simulink model "chap2_2"  (Simulink 3.00)
settings: Solver=ode45  StartTime=0.0  StopTime=10.0  RelTol=1e-3
libraries: simulink3 x1, simulink_extras x1

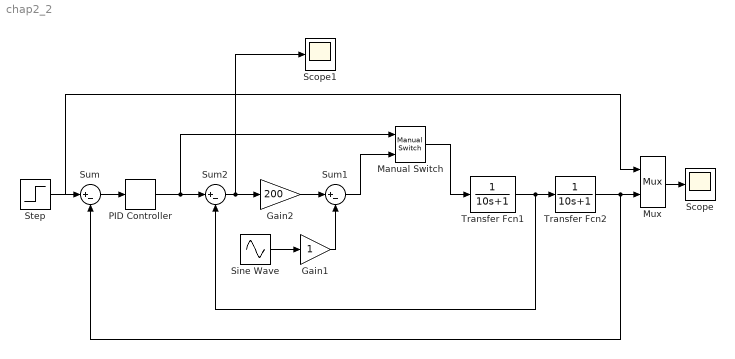
== system chap2_2 ==
  Gain1 : Gain  Gain=1  SaturateOnIntegerOverflow=on
  Gain2 : Gain  Gain=200  SaturateOnIntegerOverflow=on
  Manual Switch : simulink3/Nonlinear/Manual Switch  sw=0  action=0
  Mux : Mux  Inputs=2
      settings: DisplayOption=none
  PID Controller : simulink_extras/Additional Linear/PID Controller  P=50  I=5  D=0
  Scope : Scope
      settings: TimeRange=auto  YMin=-0.1  YMax=1  SaveToWorkspace=off  SaveName=ScopeData
  Scope1 : Scope
      settings: TimeRange=auto  YMin=-0.1  YMax=1  SaveToWorkspace=off  SaveName=ScopeData
  Sine Wave : Sin  Amplitude=1  Frequency=50  Phase=0  SampleTime=0
  Step : Step  Time=0  Before=0  After=1  SampleTime=0
  Sum : Sum  Inputs=|+-  SaturateOnIntegerOverflow=on
  Sum1 : Sum  Inputs=|+-  SaturateOnIntegerOverflow=on
  Sum2 : Sum  Inputs=|+-  SaturateOnIntegerOverflow=on
  Transfer Fcn1 : TransferFcn  Numerator=[1]  Denominator=[10 1]
  Transfer Fcn2 : TransferFcn  Numerator=[1]  Denominator=[10 1]
  wires:
  Mux/1 -> Scope/1
  Sum/1 -> PID Controller/1
  Step/1 -> Sum/1, Mux/1
  Manual Switch/1 -> Transfer Fcn1/1
  Sum1/1 -> Manual Switch/2
  Sine Wave/1 -> Gain1/1
  Gain1/1 -> Sum1/2
  Gain2/1 -> Sum1/1
  PID Controller/1 -> Sum2/1, Manual Switch/1
  Transfer Fcn1/1 -> Sum2/2, Transfer Fcn2/1
  Transfer Fcn2/1 -> Mux/2, Sum/2
  Sum2/1 -> Gain2/1, Scope1/1
